simulink model "AW_test"  (R2016b)
settings: Solver=ode8  StartTime=0.0  StopTime=0.5  FixedStep=1e-4  MaxStep=1e-4  RelTol=1e-3  EnableMultiTasking=on
values from neighbouring files (symbols this model uses):
  Ac = [-315.096994309 -3878.89771101 -17.0292118566 21.2098569883 246.813546014 484.691837637 -149.63417576 -492.819462299 3167.4151908 -130.626932997 -31.9727283183 -412.323742278 ... (144 elements, 12x12)]    [controller.mat]    (also in main_matlab_single_step.m = rlqg.A)
  Ap = A    [main_matlab_single_step.m]    (also in plant.mat = [-12.4193466298 -4275.94904034 0 0 0 0 0 0 0 0 0 0 ... (144 )
  Bcy = [-0.00424098668828 0.00299188088287 -0.110971716586 -0.350675357795 -0.314262808957 0.267697856405 -10.0334333049 -9.39488290887 0.852384232314 -56.5067664404 -23.4639342577 -28.187233595]    [controller.mat]    (also in main_matlab_single_step.m = rlqg.B)
  Bp = B    [main_matlab_single_step.m]
  Cc = [-247.527908345 97.8275933894 272.025102929 -165.96639153 4.4095489734 -129.340374453 -144.603576366 -212.735555333 46.3002432612 -57.7195976838 55.0038517645 -189.155831414 ... (24 elements, 2x12)]    [controller.mat]    (also in main_matlab_single_step.m = rlqg.C)
  Cp = C    [main_matlab_single_step.m]
  Dcy = [0 0]    [controller.mat]    (also in main_matlab_single_step.m = rlqg.D)
  GAMA1 = GAMA(1:naw,1:naw)    [main_matlab_single_step.m]
  GAMA2 = GAMA(1:naw,naw+1:end)    [main_matlab_single_step.m]
  GAMA3 = GAMA(naw+1:end,1:naw)    [main_matlab_single_step.m]
  GAMA4 = GAMA(naw+1:end,naw+1:end)    [main_matlab_single_step.m]
  Hp = H    [main_matlab_single_step.m]
  m = numel(B)/np    [main_matlab_single_step.m]
  nc = sqrt(numel(Ac))    [main_matlab_single_step.m]
libraries: fuzblock x2
settings Model: Creator=p4wp4w  LastModifiedBy=ABLAH
settings DataIOCC: LimitDataPoints=on  SaveFormat=Array
settings OptimizationCC: LifeSpan=inf
settings DebuggingCC: SFUnexpectedBacktrackingDiag=warning  SFNoUnconditionalDefaultTransitionDiag=warning  SFExecutionAtInitializationDiag=none
settings HardwareCC: ProdBitPerPointer=32  ProdBitPerSizeT=32  ProdBitPerPtrDiffT=32  ProdLargestAtomicFloat=None  ProdIntDivRoundTo=Undefined  ProdEndianess=Unspecified  ProdWordSize=32  ProdHWDeviceType=32-bit Generic
settings ModelReferenceCC: PropagateSignalLabelsOutOfModel=off
settings GRTTargetCC: TargetLangStandard=C89/C90 (ANSI)  GeneratePreprocessorConditionals=Disable all
settings ConfigComp: CovMetricSettings=dw  CovHtmlReporting=on  CovSaveCumulativeToWorkspaceVar=on  CovSaveSingleToWorkspaceVar=on  CovExternalEMLEnable=off

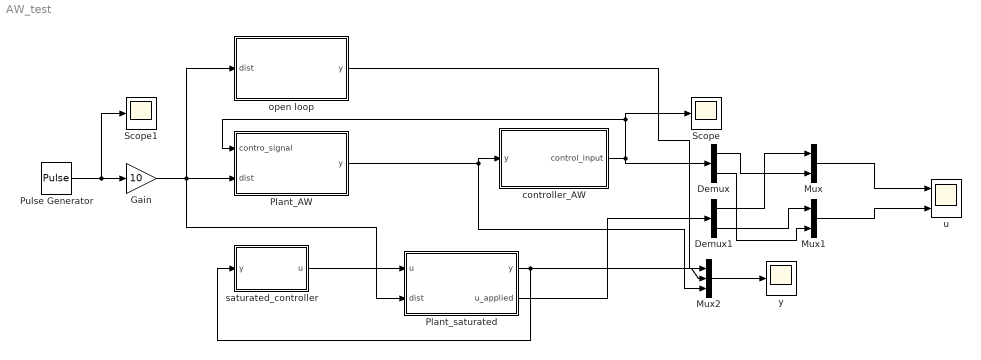
== system AW_test ==
  Demux : Demux  Outputs=2
  Demux1 : Demux  Outputs=2
  Gain : Gain  Gain=10
  Mux : Mux  Inputs=2
  Mux1 : Mux  Inputs=2
  Mux2 : Mux  Inputs=3
  Plant_AW : Subsystem
  Plant_saturated : Subsystem
  Pulse Generator : DiscretePulseGenerator  PulseType=Time based  Period=0.5  PulseWidth=10
  Scope : Scope
  Scope1 : Scope
  controller_AW : Subsystem
  open loop : Subsystem
  "saturated_controller " : Subsystem
  u : Scope  NumInputPorts=2
  y : Scope
  wires:
  Plant_AW/1(y) -> controller_AW/1(y), Mux2/3
  controller_AW/1("control_input ") -> Scope/1, Plant_AW/1(contro_signal), Demux/1
  Pulse Generator/1 -> Scope1/1, Gain/1
  "saturated_controller "/1(u) -> Plant_saturated/1(u)
  Plant_saturated/1(y) -> Mux2/2, "saturated_controller "/1(y)
  Demux1/1 -> Mux/1
  Demux/1 -> Mux/2
  Demux1/2 -> Mux1/1
  Demux/2 -> Mux1/2
  Mux/1 -> u/1
  Mux1/1 -> u/2
  Plant_saturated/2(u_applied) -> Demux1/1
  Gain/1 -> Plant_saturated/2(dist), open loop/1(dist), Plant_AW/2(dist)
  Mux2/1 -> y/1
  open loop/1(y) -> Mux2/1

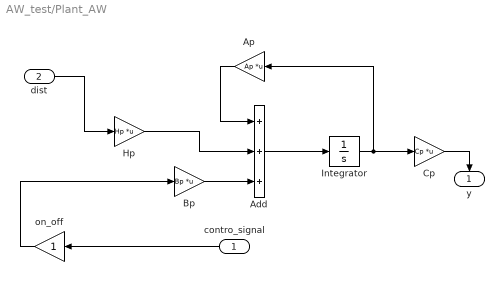
== system AW_test/Plant_AW ==
  contro_signal : Inport
  dist : Inport  Port=2
  Add : Sum  Inputs=+++
  Ap : Gain  Gain=Ap  Multiplication=Matrix(K*u)
  Bp : Gain  Gain=Bp  Multiplication=Matrix(K*u)
  Cp : Gain  Gain=Cp  Multiplication=Matrix(K*u)
  Hp : Gain  Gain=Hp  Multiplication=Matrix(K*u)
  Integrator : Integrator
  on_off : Gain
  y : Outport
  wires:
  Add/1 -> Integrator/1
  Cp/1 -> y/1
  Hp/1 -> Add/2
  on_off/1 -> Bp/1
  Integrator/1 -> Cp/1, Ap/1
  Ap/1 -> Add/1
  Bp/1 -> Add/3
  dist/1 -> Hp/1
  contro_signal/1 -> on_off/1

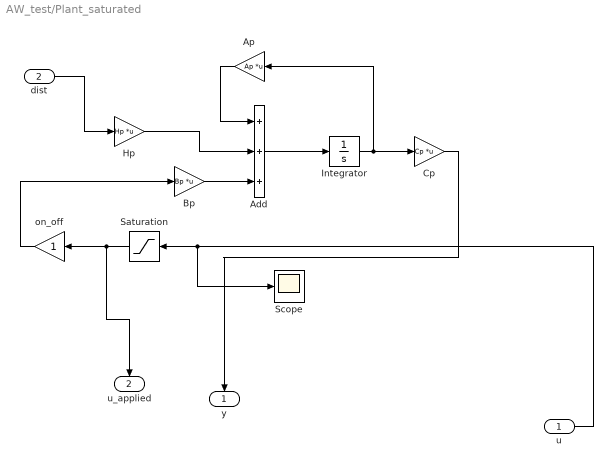
== system AW_test/Plant_saturated ==
  u : Inport
  dist : Inport  Port=2
  Add : Sum  Inputs=+++
  Ap : Gain  Gain=Ap  Multiplication=Matrix(K*u)
  Bp : Gain  Gain=Bp  Multiplication=Matrix(K*u)
  Cp : Gain  Gain=Cp  Multiplication=Matrix(K*u)
  Hp : Gain  Gain=Hp  Multiplication=Matrix(K*u)
  Integrator : Integrator
  Saturation : Saturate  UpperLimit=1.8  LowerLimit=-1.8
  Scope : Scope
  on_off : Gain
  y : Outport
  u_applied : Outport  Port=2
  wires:
  dist/1 -> Hp/1
  Bp/1 -> Add/3
  u/1 -> Scope/1, Saturation/1
  Ap/1 -> Add/1
  Saturation/1 -> u_applied/1, on_off/1
  Integrator/1 -> Ap/1, Cp/1
  on_off/1 -> Bp/1
  Hp/1 -> Add/2
  Cp/1 -> y/1
  Add/1 -> Integrator/1

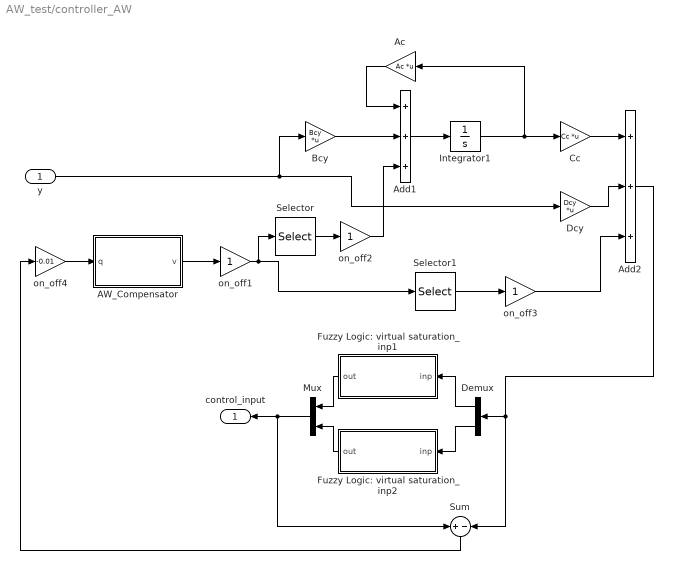
== system AW_test/controller_AW ==
  y : Inport
  AW_Compensator : Subsystem
  Ac : Gain  Gain=Ac  Multiplication=Matrix(K*u)
  Add1 : Sum  Inputs=+++
  Add2 : Sum  Inputs=+++
  Bcy : Gain  Gain=Bcy  Multiplication=Matrix(K*u)
  Cc : Gain  Gain=Cc  Multiplication=Matrix(K*u)
  Dcy : Gain  Gain=Dcy  Multiplication=Matrix(K*u)
  Demux : Demux  Outputs=2
  Fuzzy Logic: virtual saturation_inp1 : Subsystem
  Fuzzy Logic: virtual saturation_inp2 : Subsystem
  Integrator1 : Integrator
  Mux : Mux  Inputs=2
  Selector : Selector  InputPortWidth=nc+m  IndexOptions=Index vector (dialog)  Indices=[1:nc]  OutputSizes=1
  Selector1 : Selector  InputPortWidth=nc+m  IndexOptions=Index vector (dialog)  Indices=[nc+1:nc+m]  OutputSizes=1
  Sum : Sum  Inputs=+|-
  on_off1 : Gain
  on_off2 : Gain
  on_off3 : Gain
  on_off4 : Gain  Gain=-0.01
  "control_input " : Outport
  wires:
  Cc/1 -> Add2/1
  Add1/1 -> Integrator1/1
  Ac/1 -> Add1/1
  AW_Compensator/1(v) -> on_off1/1
  Bcy/1 -> Add1/2
  Integrator1/1 -> Cc/1, Ac/1
  Dcy/1 -> Add2/2
  y/1 -> Dcy/1, Bcy/1
  Sum/1 -> on_off4/1
  on_off2/1 -> Add1/3
  on_off3/1 -> Add2/3
  Selector1/1 -> on_off3/1
  on_off1/1 -> Selector/1, Selector1/1
  Selector/1 -> on_off2/1
  on_off4/1 -> AW_Compensator/1(q)
  Fuzzy Logic: virtual saturation_inp1/1(out) -> Mux/1
  Fuzzy Logic: virtual saturation_inp2/1(out) -> Mux/2
  Mux/1 -> Sum/1, "control_input "/1
  Demux/2 -> Fuzzy Logic: virtual saturation_inp2/1(inp)
  Demux/1 -> Fuzzy Logic: virtual saturation_inp1/1(inp)
  Add2/1 -> Demux/1, Sum/2

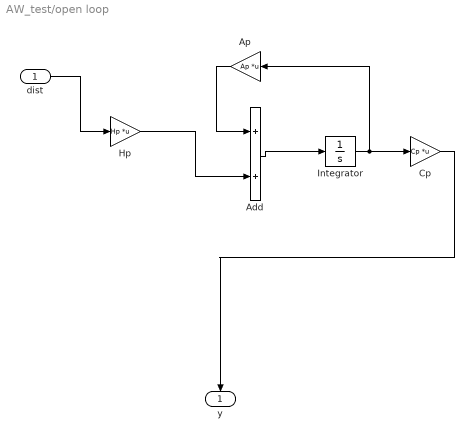
== system AW_test/open loop ==
  dist : Inport
  Add : Sum
  Ap : Gain  Gain=Ap  Multiplication=Matrix(K*u)
  Cp : Gain  Gain=Cp  Multiplication=Matrix(K*u)
  Hp : Gain  Gain=Hp  Multiplication=Matrix(K*u)
  Integrator : Integrator
  y : Outport
  wires:
  dist/1 -> Hp/1
  Ap/1 -> Add/1
  Integrator/1 -> Ap/1, Cp/1
  Hp/1 -> Add/2
  Cp/1 -> y/1
  Add/1 -> Integrator/1

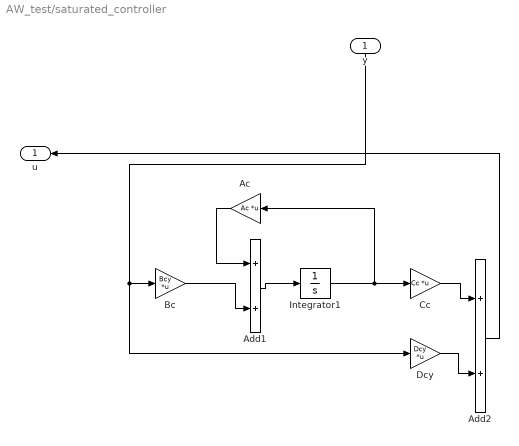
== system AW_test/saturated_controller  ==
  y : Inport
  Ac : Gain  Gain=Ac  Multiplication=Matrix(K*u)
  Add1 : Sum
  Add2 : Sum
  Bc : Gain  Gain=Bcy  Multiplication=Matrix(K*u)
  Cc : Gain  Gain=Cc  Multiplication=Matrix(K*u)
  Dcy : Gain  Gain=Dcy  Multiplication=Matrix(K*u)
  Integrator1 : Integrator
  u : Outport
  wires:
  Bc/1 -> Add1/2
  Add1/1 -> Integrator1/1
  Cc/1 -> Add2/1
  Dcy/1 -> Add2/2
  Integrator1/1 -> Cc/1, Ac/1
  Add2/1 -> u/1
  Ac/1 -> Add1/1
  y/1 -> Bc/1, Dcy/1

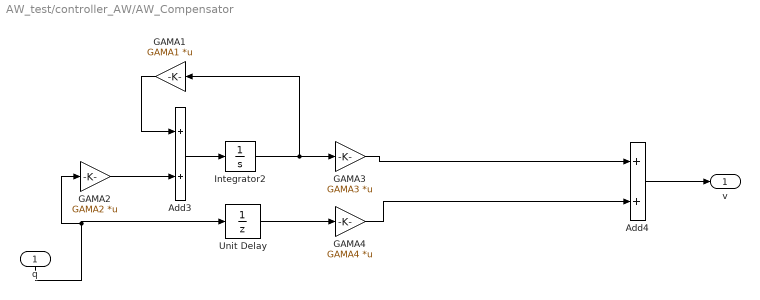
== system AW_test/controller_AW/AW_Compensator ==
  q : Inport
  Add3 : Sum
  Add4 : Sum
  GAMA1 : Gain  Gain=GAMA1  Multiplication=Matrix(K*u)
  GAMA2 : Gain  Gain=GAMA2  Multiplication=Matrix(K*u)
  GAMA3 : Gain  Gain=GAMA3  Multiplication=Matrix(K*u)
  GAMA4 : Gain  Gain=GAMA4  Multiplication=Matrix(K*u)
  Integrator2 : Integrator
  Unit Delay : UnitDelay  SampleTime=-1
  v : Outport
  wires:
  Add3/1 -> Integrator2/1
  GAMA3/1 -> Add4/1
  GAMA1/1 -> Add3/1
  Integrator2/1 -> GAMA1/1, GAMA3/1
  GAMA2/1 -> Add3/2
  GAMA4/1 -> Add4/2
  Add4/1 -> v/1
  q/1 -> Unit Delay/1, GAMA2/1
  Unit Delay/1 -> GAMA4/1

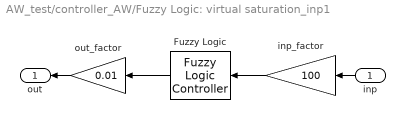
== system AW_test/controller_AW/Fuzzy Logic: virtual saturation_inp1 ==
  inp : Inport
  Fuzzy Logic : fuzblock/Fuzzy Logic  Controller  fis='FSMO.fis'
  inp_factor : Gain  Gain=100
  out_factor : Gain  Gain=0.01
  out : Outport
  wires:
  inp_factor/1 -> Fuzzy Logic/1
  out_factor/1 -> out/1
  inp/1 -> inp_factor/1
  Fuzzy Logic/1 -> out_factor/1

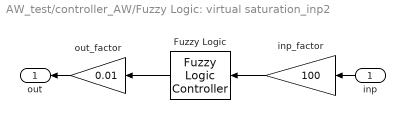
== system AW_test/controller_AW/Fuzzy Logic: virtual saturation_inp2 ==
  inp : Inport
  Fuzzy Logic : fuzblock/Fuzzy Logic  Controller  fis='FSMO.fis'
  inp_factor : Gain  Gain=100
  out_factor : Gain  Gain=0.01
  out : Outport
  wires:
  Fuzzy Logic/1 -> out_factor/1
  inp/1 -> inp_factor/1
  out_factor/1 -> out/1
  inp_factor/1 -> Fuzzy Logic/1
